simulink model "robust_trajectory"  (R2024b)
settings: Solver=VariableStepAuto  StartTime=0.0  StopTime=10.0  RelTol=1e-3
settings Model: Creator=johnn  LastModifiedBy=johnn

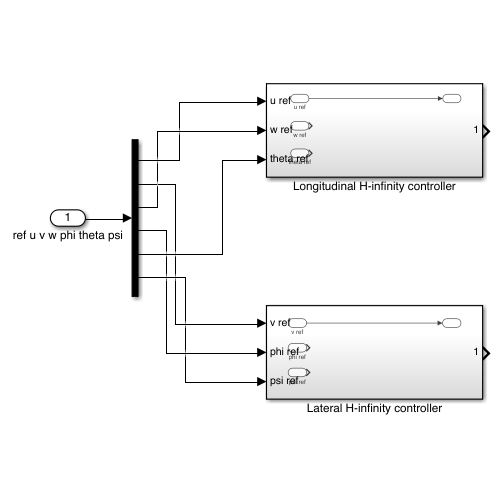
[thumbnail: Simulink's stored preview of the top-level diagram]
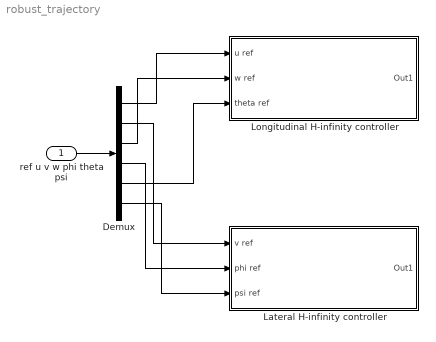
== system robust_trajectory ==
  ref u v w phi theta psi : Inport
  Demux : Demux  Outputs=6
  Lateral H-infinity controller : Subsystem
  Longitudinal H-infinity controller : Subsystem
  wires:
  ref u v w phi theta psi/1 -> Demux/1
  Demux/1 -> Longitudinal H-infinity controller/1(u ref)
  Demux/2 -> Lateral H-infinity controller/1(v ref)
  Demux/3 -> Longitudinal H-infinity controller/2(w ref)
  Demux/4 -> Lateral H-infinity controller/2(phi ref)
  Demux/5 -> Longitudinal H-infinity controller/3(theta ref)
  Demux/6 -> Lateral H-infinity controller/3(psi ref)

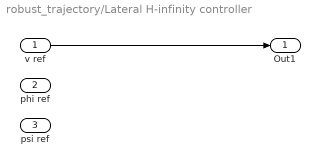
== system robust_trajectory/Lateral H-infinity controller ==
  v ref : Inport
  phi ref : Inport  Port=2
  psi ref : Inport  Port=3
  Out1 : Outport
  wires:
  v ref/1 -> Out1/1

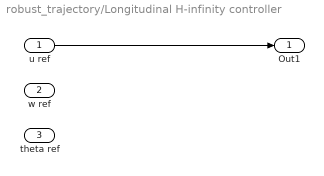
== system robust_trajectory/Longitudinal H-infinity controller ==
  u ref : Inport
  w ref : Inport  Port=2
  theta ref : Inport  Port=3
  Out1 : Outport
  wires:
  u ref/1 -> Out1/1
